simulink model "AirbagModel"  (Simulink 8.5)
settings: Solver=ode1  StartTime=0.0  StopTime=10.0  RelTol=1e-3
libraries: simulink x1
settings Model: Creator=gwilli10  LastModifiedBy=jonah.caplan  CovSFcnEnable=off
settings DataIOCC: SignalLoggingSaveFormat=Dataset
settings OptimizationCC: ExpressionDepthLimit=128  OptimizeModelRefInitCode=on  LifeSpan=1
settings DebuggingCC: UnderspecifiedInitializationDetection=Simplified  MergeDetectMultiDrivingBlocksExec=error  SolverPrmCheckMsg=warning  FcnCallInpInsideContextMsg=EnableAllAsError  StateNameClashWarn=none
settings HardwareCC: ProdIntDivRoundTo=Floor  ProdEndianess=LittleEndian  ProdHWDeviceType=Generic->32-bit Embedded Processor  TargetEndianess=LittleEndian  TargetHWDeviceType=Generic->32-bit Embedded Processor
settings RTWCC: SystemTargetFile=ert.tlc  GenCodeOnly=on  TemplateMakefile=ert_default_tmf  Description=Embedded Coder
settings CodeAppCC: IgnoreCustomStorageClasses=off  MATLABSourceComments=on
settings ERTTargetCC: MultiwordLength=2048  GenerateSampleERTMain=on  MultiInstanceERTCode=on  CodeInterfacePackaging=Reusable function  RootIOFormat=Structure reference  ERTCustomFileTemplate=example_file_process.tlc  GlobalDataDefinition=InSeparateSourceFile  GlobalDataReference=InSeparateHeaderFile  ERTFilePackagingFormat=CompactWithDataFile  SuppressUnreachableDefaultCases=off

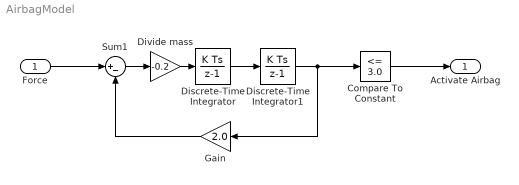
== system AirbagModel ==
  Force : Inport
  Compare To Constant : simulink/Logic and Bit Operations/Compare To Constant  relop=<=  const=3.0  OutDataTypeStr=boolean
  Discrete-Time Integrator : DiscreteIntegrator
  Discrete-Time Integrator1 : DiscreteIntegrator
  Divide mass : Gain  Gain=-0.2
  Gain : Gain  Gain=2.0
  Sum1 : Sum  Inputs=|+-
  "Activate Airbag " : Outport
  wires:
  Discrete-Time Integrator1/1 -> Compare To Constant/1, Gain/1
  Gain/1 -> Sum1/2
  Sum1/1 -> Divide mass/1
  Divide mass/1 -> Discrete-Time Integrator/1
  Force/1 -> Sum1/1
  Discrete-Time Integrator/1 -> Discrete-Time Integrator1/1
  Compare To Constant/1 -> "Activate Airbag "/1
